simulink model "spe_servomotor_mod"  (R2019a)
settings: Solver=ode23t  StartTime=0.0  StopTime=5  FixedStep=0.001  RelTol=1e-4  EnableMultiTasking=on
model workspace (MAT data in the model file):
  B = 0.000415543589544
  J = 9.65688521823e-08
  Jd = 0.000158042874485
  Km = 0.0648451554932
  La = 0.00823160993738
  Ra = 0.292898808666
  spe_servomotor_mod_spesession : sldodialogs.data.SessionData (value not decoded)
  spe_servomotor_sdosession = sldodialogs.data.SessionData
  spe_servomotor_sdosession.Version = '3.0'
  spe_servomotor_sdosession.Data.ModelName = 'spe_servomotor'
  spe_servomotor_sdosession.Data.ToolType = 'ParameterEstimation'
  spe_servomotor_sdosession.Data.GUIOptions.NoPromptClose = 0
  spe_servomotor_sdosession.Data.Workspace.LocalWorkspace.EstimationData = sdo.Experiment
  spe_servomotor_sdosession.Data.Workspace.LocalWorkspace.EstimationData.ModelName = 'spe_servomotor'
  spe_servomotor_sdosession.Data.Workspace.LocalWorkspace.EstimationData.InputData = Simulink.SimulationData.Signal
  spe_servomotor_sdosession.Data.Workspace.LocalWorkspace.EstimationData.InputData.BlockPath = Simulink.SimulationData.BlockPath
  spe_servomotor_sdosession.Data.Workspace.LocalWorkspace.EstimationData.InputData.BlockPath.path = {'spe_servomotor/Input Signal (V)'}
  spe_servomotor_sdosession.Data.Workspace.LocalWorkspace.EstimationData.InputData.Values = timeseries
  spe_servomotor_sdosession.Data.Workspace.LocalWorkspace.EstimationData.InputData.Values.Name = 'spe_servomotor/Input Signal (V):1'
  spe_servomotor_sdosession.Data.Workspace.LocalWorkspace.EstimationData.InputData.Values.DataInfo = tsdata.datametadata
  spe_servomotor_sdosession.Data.Workspace.LocalWorkspace.EstimationData.InputData.Values.DataInfo.Interpolation = tsdata.interpolation
  spe_servomotor_sdosession.Data.Workspace.LocalWorkspace.EstimationData.InputData.Values.DataInfo.Interpolation.Fhandle : function handle (value not decoded)
  spe_servomotor_sdosession.Data.Workspace.LocalWorkspace.EstimationData.InputData.Values.DataInfo.Interpolation.Name = 'linear'
  spe_servomotor_sdosession.Data.Workspace.LocalWorkspace.EstimationData.InputData.Values.TimeInfo = tsdata.timemetadata
  spe_servomotor_sdosession.Data.Workspace.LocalWorkspace.EstimationData.InputData.Values.TimeInfo.Length = 1001
  spe_servomotor_sdosession.Data.Workspace.LocalWorkspace.EstimationData.InputData.Values.TimeInfo.DuplicateTimes = 0
  spe_servomotor_sdosession.Data.Workspace.LocalWorkspace.EstimationData.InputData.Values.TimeInfo.Time_ = [0 0.005 0.01 0.015 0.02 0.025 0.03 0.035 0.04 0.045 0.05 0.055 ... (1001 elements, 1001x1)]
  spe_servomotor_sdosession.Data.Workspace.LocalWorkspace.EstimationData.InputData.Values.TimeInfo.Initialized = 1
  spe_servomotor_sdosession.Data.Workspace.LocalWorkspace.EstimationData.InputData.Values.QualityInfo = tsdata.qualmetadata
  spe_servomotor_sdosession.Data.Workspace.LocalWorkspace.EstimationData.InputData.Values.Data_ = [1 1 1 1 1 1 1 1 1 1 1 1 ... (1001 elements, 1001x1)]
  spe_servomotor_sdosession.Data.Workspace.LocalWorkspace.EstimationData.InputData.Name = 'spe_servomotor/Input Signal (V):1'
  spe_servomotor_sdosession.Data.Workspace.LocalWorkspace.EstimationData.OutputData = Simulink.SimulationData.Signal
  spe_servomotor_sdosession.Data.Workspace.LocalWorkspace.EstimationData.OutputData.PortType = 'outport'
  spe_servomotor_sdosession.Data.Workspace.LocalWorkspace.EstimationData.OutputData.BlockPath = Simulink.SimulationData.BlockPath
  spe_servomotor_sdosession.Data.Workspace.LocalWorkspace.EstimationData.OutputData.BlockPath.path = {'spe_servomotor/rad to deg'}
  spe_servomotor_sdosession.Data.Workspace.LocalWorkspace.EstimationData.OutputData.Values = timeseries
  spe_servomotor_sdosession.Data.Workspace.LocalWorkspace.EstimationData.OutputData.Values.Name = 'spe_servomotor/rad to deg:1'
  spe_servomotor_sdosession.Data.Workspace.LocalWorkspace.EstimationData.OutputData.Values.DataInfo = tsdata.datametadata
  spe_servomotor_sdosession.Data.Workspace.LocalWorkspace.EstimationData.OutputData.Values.DataInfo.Interpolation = tsdata.interpolation
  spe_servomotor_sdosession.Data.Workspace.LocalWorkspace.EstimationData.OutputData.Values.DataInfo.Interpolation.Fhandle : function handle (value not decoded)
  spe_servomotor_sdosession.Data.Workspace.LocalWorkspace.EstimationData.OutputData.Values.DataInfo.Interpolation.Name = 'linear'
  spe_servomotor_sdosession.Data.Workspace.LocalWorkspace.EstimationData.OutputData.Values.TimeInfo = tsdata.timemetadata
  spe_servomotor_sdosession.Data.Workspace.LocalWorkspace.EstimationData.OutputData.Values.TimeInfo.Length = 1001
  spe_servomotor_sdosession.Data.Workspace.LocalWorkspace.EstimationData.OutputData.Values.TimeInfo.DuplicateTimes = 0
  spe_servomotor_sdosession.Data.Workspace.LocalWorkspace.EstimationData.OutputData.Values.TimeInfo.Time_ = [0 0.005 0.01 0.015 0.02 0.025 0.03 0.035 0.04 0.045 0.05 0.055 ... (1001 elements, 1001x1)]
  spe_servomotor_sdosession.Data.Workspace.LocalWorkspace.EstimationData.OutputData.Values.TimeInfo.Initialized = 1
  spe_servomotor_sdosession.Data.Workspace.LocalWorkspace.EstimationData.OutputData.Values.QualityInfo = tsdata.qualmetadata
  spe_servomotor_sdosession.Data.Workspace.LocalWorkspace.EstimationData.OutputData.Values.Data_ = [2.64853348517 2.69948102795 2.8809816491 3.35224641981 3.98272226171 4.71827741059 5.33283214537 6.22441414402 7.17012790686 7.9534463771 8.97239723269 9.90855833127 ... (1001 elements, 1001x1)]
  spe_servomotor_sdosession.Data.Workspace.LocalWorkspace.EstimationData.OutputData.Name = 'spe_servomotor/rad to deg:1'
  spe_servomotor_sdosession.Data.Workspace.LocalWorkspace.EstimationData.Name = 'EstimationData'
  spe_servomotor_sdosession.Data.Workspace.LocalWorkspace.ValidationData = sdo.Experiment
  spe_servomotor_sdosession.Data.Workspace.LocalWorkspace.ValidationData.ModelName = 'spe_servomotor'
  spe_servomotor_sdosession.Data.Workspace.LocalWorkspace.ValidationData.InputData = Simulink.SimulationData.Signal
  spe_servomotor_sdosession.Data.Workspace.LocalWorkspace.ValidationData.InputData.BlockPath = Simulink.SimulationData.BlockPath
  spe_servomotor_sdosession.Data.Workspace.LocalWorkspace.ValidationData.InputData.BlockPath.path = {'spe_servomotor/Input Signal (V)'}
  spe_servomotor_sdosession.Data.Workspace.LocalWorkspace.ValidationData.InputData.Values = timeseries
  spe_servomotor_sdosession.Data.Workspace.LocalWorkspace.ValidationData.InputData.Values.Name = 'unnamed'
  spe_servomotor_sdosession.Data.Workspace.LocalWorkspace.ValidationData.InputData.Values.DataInfo = tsdata.datametadata
  spe_servomotor_sdosession.Data.Workspace.LocalWorkspace.ValidationData.InputData.Values.DataInfo.Interpolation = tsdata.interpolation
  spe_servomotor_sdosession.Data.Workspace.LocalWorkspace.ValidationData.InputData.Values.DataInfo.Interpolation.Fhandle : function handle (value not decoded)
  spe_servomotor_sdosession.Data.Workspace.LocalWorkspace.ValidationData.InputData.Values.DataInfo.Interpolation.Name = 'linear'
  spe_servomotor_sdosession.Data.Workspace.LocalWorkspace.ValidationData.InputData.Values.TimeInfo = tsdata.timemetadata
  spe_servomotor_sdosession.Data.Workspace.LocalWorkspace.ValidationData.InputData.Values.TimeInfo.Length = 1001
  spe_servomotor_sdosession.Data.Workspace.LocalWorkspace.ValidationData.InputData.Values.TimeInfo.DuplicateTimes = 0
  spe_servomotor_sdosession.Data.Workspace.LocalWorkspace.ValidationData.InputData.Values.TimeInfo.Time_ = [0 0.005 0.01 0.015 0.02 0.025 0.03 0.035 0.04 0.045 0.05 0.055 ... (1001 elements, 1001x1)]
  spe_servomotor_sdosession.Data.Workspace.LocalWorkspace.ValidationData.InputData.Values.TimeInfo.Initialized = 1
  spe_servomotor_sdosession.Data.Workspace.LocalWorkspace.ValidationData.InputData.Values.QualityInfo = tsdata.qualmetadata
  spe_servomotor_sdosession.Data.Workspace.LocalWorkspace.ValidationData.InputData.Values.Data_ = [0 0 0 0 0 0 0 0 0 0 0 0 ... (1001 elements, 1001x1)]
  spe_servomotor_sdosession.Data.Workspace.LocalWorkspace.ValidationData.OutputData = Simulink.SimulationData.Signal
  spe_servomotor_sdosession.Data.Workspace.LocalWorkspace.ValidationData.OutputData.PortType = 'outport'
  spe_servomotor_sdosession.Data.Workspace.LocalWorkspace.ValidationData.OutputData.BlockPath = Simulink.SimulationData.BlockPath
  spe_servomotor_sdosession.Data.Workspace.LocalWorkspace.ValidationData.OutputData.BlockPath.path = {'spe_servomotor/rad to deg'}
  spe_servomotor_sdosession.Data.Workspace.LocalWorkspace.ValidationData.OutputData.Values = timeseries
  spe_servomotor_sdosession.Data.Workspace.LocalWorkspace.ValidationData.OutputData.Values.Name = 'unnamed'
  spe_servomotor_sdosession.Data.Workspace.LocalWorkspace.ValidationData.OutputData.Values.DataInfo = tsdata.datametadata
  spe_servomotor_sdosession.Data.Workspace.LocalWorkspace.ValidationData.OutputData.Values.DataInfo.Interpolation = tsdata.interpolation
  spe_servomotor_sdosession.Data.Workspace.LocalWorkspace.ValidationData.OutputData.Values.DataInfo.Interpolation.Fhandle : function handle (value not decoded)
  spe_servomotor_sdosession.Data.Workspace.LocalWorkspace.ValidationData.OutputData.Values.DataInfo.Interpolation.Name = 'linear'
  spe_servomotor_sdosession.Data.Workspace.LocalWorkspace.ValidationData.OutputData.Values.TimeInfo = tsdata.timemetadata
  spe_servomotor_sdosession.Data.Workspace.LocalWorkspace.ValidationData.OutputData.Values.TimeInfo.Length = 1001
  spe_servomotor_sdosession.Data.Workspace.LocalWorkspace.ValidationData.OutputData.Values.TimeInfo.DuplicateTimes = 0
  spe_servomotor_sdosession.Data.Workspace.LocalWorkspace.ValidationData.OutputData.Values.TimeInfo.Time_ = [0 0.005 0.01 0.015 0.02 0.025 0.03 0.035 0.04 0.045 0.05 0.055 ... (1001 elements, 1001x1)]
  spe_servomotor_sdosession.Data.Workspace.LocalWorkspace.ValidationData.OutputData.Values.TimeInfo.Initialized = 1
  spe_servomotor_sdosession.Data.Workspace.LocalWorkspace.ValidationData.OutputData.Values.QualityInfo = tsdata.qualmetadata
  spe_servomotor_sdosession.Data.Workspace.LocalWorkspace.ValidationData.OutputData.Values.Data_ = [2.6485 2.6485 2.64849999999 2.64849999999 2.64849999999 2.64849999999 2.64849999999 2.64849999999 2.64849999999 2.64849999999 2.64849999999 2.64849999999 ... (1001 elements, 1001x1)]
  spe_servomotor_sdosession.Data.Workspace.LocalWorkspace.ValidationData.Name = 'ValidationData'
  spe_servomotor_sdosession.Data.Workspace.HiddenWorkspace.EstimatedParams(1) = param.Continuous
  spe_servomotor_sdosession.Data.Workspace.HiddenWorkspace.EstimatedParams(1).Minimum_ = 0
  spe_servomotor_sdosession.Data.Workspace.HiddenWorkspace.EstimatedParams(1).Scale_ = 0.008
  spe_servomotor_sdosession.Data.Workspace.HiddenWorkspace.EstimatedParams(1).Size_ = [1 1]
  spe_servomotor_sdosession.Data.Workspace.HiddenWorkspace.EstimatedParams(1).Value_ = 0.008
  spe_servomotor_sdosession.Data.Workspace.HiddenWorkspace.EstimatedParams(1).pID = paramid.Variable
  spe_servomotor_sdosession.Data.Workspace.HiddenWorkspace.EstimatedParams(1).pID.Name = 'B'
  spe_servomotor_sdosession.Data.Workspace.HiddenWorkspace.EstimatedParams(2) = param.Continuous
  spe_servomotor_sdosession.Data.Workspace.HiddenWorkspace.EstimatedParams(2).Minimum_ = 0
  spe_servomotor_sdosession.Data.Workspace.HiddenWorkspace.EstimatedParams(2).Scale_ = 5.7e-07
  spe_servomotor_sdosession.Data.Workspace.HiddenWorkspace.EstimatedParams(2).Size_ = [1 1]
  spe_servomotor_sdosession.Data.Workspace.HiddenWorkspace.EstimatedParams(2).Value_ = 5.7e-07
  spe_servomotor_sdosession.Data.Workspace.HiddenWorkspace.EstimatedParams(2).pID = paramid.Variable
  spe_servomotor_sdosession.Data.Workspace.HiddenWorkspace.EstimatedParams(2).pID.Name = 'J'
  spe_servomotor_sdosession.Data.Workspace.HiddenWorkspace.EstimatedParams(3) = param.Continuous
  spe_servomotor_sdosession.Data.Workspace.HiddenWorkspace.EstimatedParams(3).Minimum_ = 0
  spe_servomotor_sdosession.Data.Workspace.HiddenWorkspace.EstimatedParams(3).Scale_ = 0.0134
  spe_servomotor_sdosession.Data.Workspace.HiddenWorkspace.EstimatedParams(3).Size_ = [1 1]
  spe_servomotor_sdosession.Data.Workspace.HiddenWorkspace.EstimatedParams(3).Value_ = 0.0134
  spe_servomotor_sdosession.Data.Workspace.HiddenWorkspace.EstimatedParams(3).pID = paramid.Variable
  spe_servomotor_sdosession.Data.Workspace.HiddenWorkspace.EstimatedParams(3).pID.Name = 'Km'
  spe_servomotor_sdosession.Data.Workspace.HiddenWorkspace.EstimatedParams(4) = param.Continuous
  spe_servomotor_sdosession.Data.Workspace.HiddenWorkspace.EstimatedParams(4).Minimum_ = 0
  spe_servomotor_sdosession.Data.Workspace.HiddenWorkspace.EstimatedParams(4).Scale_ = 6.5e-05
  spe_servomotor_sdosession.Data.Workspace.HiddenWorkspace.EstimatedParams(4).Size_ = [1 1]
  spe_servomotor_sdosession.Data.Workspace.HiddenWorkspace.EstimatedParams(4).Value_ = 6.5e-05
  spe_servomotor_sdosession.Data.Workspace.HiddenWorkspace.EstimatedParams(4).pID = paramid.Variable
  spe_servomotor_sdosession.Data.Workspace.HiddenWorkspace.EstimatedParams(4).pID.Name = 'La'
  spe_servomotor_sdosession.Data.Workspace.HiddenWorkspace.EstimatedParams(5) = param.Continuous
  spe_servomotor_sdosession.Data.Workspace.HiddenWorkspace.EstimatedParams(5).Minimum_ = 0
  spe_servomotor_sdosession.Data.Workspace.HiddenWorkspace.EstimatedParams(5).Scale_ = 1.9
  spe_servomotor_sdosession.Data.Workspace.HiddenWorkspace.EstimatedParams(5).Size_ = [1 1]
  spe_servomotor_sdosession.Data.Workspace.HiddenWorkspace.EstimatedParams(5).Value_ = 1.9
  spe_servomotor_sdosession.Data.Workspace.HiddenWorkspace.EstimatedParams(5).pID = paramid.Variable
  spe_servomotor_sdosession.Data.Workspace.HiddenWorkspace.EstimatedParams(5).pID.Name = 'Ra'
  spe_servomotor_sdosession.Data.Workspace.HiddenWorkspace.UVars = []
  spe_servomotor_sdosession.Data.ToolData.PlotManager.Plots.Class = 'sldoplots.ExperimentPlot'
  spe_servomotor_sdosession.Data.ToolData.PlotManager.Plots.Sources = {'EstimationData'}
  spe_servomotor_sdosession.Data.ToolData.DialogManager = []
  spe_servomotor_sdosession.Data.ToolData.ParameterEstimation.DesignVariables = 'EstimatedParams'
  spe_servomotor_sdosession.Data.ToolData.ParameterEstimation.UncertainVariables = 'UVars'
  spe_servomotor_sdosession.Data.ToolData.ParameterEstimation.Options = sdo.OptimizeOptions
  spe_servomotor_sdosession.Data.ToolData.ParameterEstimation.Options.Method = 'lsqnonlin'
  spe_servomotor_sdosession.Data.ToolData.ParameterEstimation.Options.MethodOptions.Display = 'iter'
  spe_servomotor_sdosession.Data.ToolData.ParameterEstimation.Options.MethodOptions.MaxFunEvals = 400
  spe_servomotor_sdosession.Data.ToolData.ParameterEstimation.Options.MethodOptions.MaxIter = 100
  spe_servomotor_sdosession.Data.ToolData.ParameterEstimation.Options.MethodOptions.TolFun = 0.2
  spe_servomotor_sdosession.Data.ToolData.ParameterEstimation.Options.MethodOptions.TolX = 1e-06
  spe_servomotor_sdosession.Data.ToolData.ParameterEstimation.Options.MethodOptions.FunValCheck = 'off'
  spe_servomotor_sdosession.Data.ToolData.ParameterEstimation.Options.MethodOptions.OutputFcn = []
  spe_servomotor_sdosession.Data.ToolData.ParameterEstimation.Options.MethodOptions.PlotFcns = []
  spe_servomotor_sdosession.Data.ToolData.ParameterEstimation.Options.MethodOptions.ActiveConstrTol = []
  spe_servomotor_sdosession.Data.ToolData.ParameterEstimation.Options.MethodOptions.Algorithm = 'trust-region-reflective'
  spe_servomotor_sdosession.Data.ToolData.ParameterEstimation.Options.MethodOptions.AlwaysHonorConstraints = []
  spe_servomotor_sdosession.Data.ToolData.ParameterEstimation.Options.MethodOptions.BranchStrategy = []
  spe_servomotor_sdosession.Data.ToolData.ParameterEstimation.Options.MethodOptions.DerivativeCheck = 'off'
  spe_servomotor_sdosession.Data.ToolData.ParameterEstimation.Options.MethodOptions.Diagnostics = 'off'
  spe_servomotor_sdosession.Data.ToolData.ParameterEstimation.Options.MethodOptions.DiffMaxChange = 0.1
  spe_servomotor_sdosession.Data.ToolData.ParameterEstimation.Options.MethodOptions.DiffMinChange = 1e-08
  spe_servomotor_sdosession.Data.ToolData.ParameterEstimation.Options.MethodOptions.FinDiffRelStep = []
  spe_servomotor_sdosession.Data.ToolData.ParameterEstimation.Options.MethodOptions.FinDiffType = 'forward'
  spe_servomotor_sdosession.Data.ToolData.ParameterEstimation.Options.MethodOptions.GoalsExactAchieve = []
  spe_servomotor_sdosession.Data.ToolData.ParameterEstimation.Options.MethodOptions.GradConstr = []
  spe_servomotor_sdosession.Data.ToolData.ParameterEstimation.Options.MethodOptions.GradObj = []
  spe_servomotor_sdosession.Data.ToolData.ParameterEstimation.Options.MethodOptions.HessFcn = []
  spe_servomotor_sdosession.Data.ToolData.ParameterEstimation.Options.MethodOptions.Hessian = []
  spe_servomotor_sdosession.Data.ToolData.ParameterEstimation.Options.MethodOptions.HessMult = []
  spe_servomotor_sdosession.Data.ToolData.ParameterEstimation.Options.MethodOptions.HessPattern = []
  spe_servomotor_sdosession.Data.ToolData.ParameterEstimation.Options.MethodOptions.HessUpdate = []
  spe_servomotor_sdosession.Data.ToolData.ParameterEstimation.Options.MethodOptions.InitialHessType = []
  spe_servomotor_sdosession.Data.ToolData.ParameterEstimation.Options.MethodOptions.InitialHessMatrix = []
  spe_servomotor_sdosession.Data.ToolData.ParameterEstimation.Options.MethodOptions.InitBarrierParam = []
  spe_servomotor_sdosession.Data.ToolData.ParameterEstimation.Options.MethodOptions.InitTrustRegionRadius = []
  spe_servomotor_sdosession.Data.ToolData.ParameterEstimation.Options.MethodOptions.Jacobian = 'on'
  spe_servomotor_sdosession.Data.ToolData.ParameterEstimation.Options.MethodOptions.JacobMult = []
  spe_servomotor_sdosession.Data.ToolData.ParameterEstimation.Options.MethodOptions.JacobPattern = 'sparse(ones(jrows,jcols))'
  spe_servomotor_sdosession.Data.ToolData.ParameterEstimation.Options.MethodOptions.LargeScale = []
  spe_servomotor_sdosession.Data.ToolData.ParameterEstimation.Options.MethodOptions.MaxNodes = []
  spe_servomotor_sdosession.Data.ToolData.ParameterEstimation.Options.MethodOptions.MaxPCGIter = 'max(1,floor(numberofvariables/2))'
  spe_servomotor_sdosession.Data.ToolData.ParameterEstimation.Options.MethodOptions.MaxProjCGIter = []
  spe_servomotor_sdosession.Data.ToolData.ParameterEstimation.Options.MethodOptions.MaxRLPIter = []
  spe_servomotor_sdosession.Data.ToolData.ParameterEstimation.Options.MethodOptions.MaxSQPIter = []
  spe_servomotor_sdosession.Data.ToolData.ParameterEstimation.Options.MethodOptions.MaxTime = []
  spe_servomotor_sdosession.Data.ToolData.ParameterEstimation.Options.MethodOptions.MeritFunction = []
  spe_servomotor_sdosession.Data.ToolData.ParameterEstimation.Options.MethodOptions.MinAbsMax = []
  spe_servomotor_sdosession.Data.ToolData.ParameterEstimation.Options.MethodOptions.NodeDisplayInterval = []
  spe_servomotor_sdosession.Data.ToolData.ParameterEstimation.Options.MethodOptions.NodeSearchStrategy = []
  spe_servomotor_sdosession.Data.ToolData.ParameterEstimation.Options.MethodOptions.NoStopIfFlatInfeas = []
  spe_servomotor_sdosession.Data.ToolData.ParameterEstimation.Options.MethodOptions.ObjectiveLimit = []
  spe_servomotor_sdosession.Data.ToolData.ParameterEstimation.Options.MethodOptions.PhaseOneTotalScaling = []
  spe_servomotor_sdosession.Data.ToolData.ParameterEstimation.Options.MethodOptions.Preconditioner = []
  spe_servomotor_sdosession.Data.ToolData.ParameterEstimation.Options.MethodOptions.PrecondBandWidth = Inf
  spe_servomotor_sdosession.Data.ToolData.ParameterEstimation.Options.MethodOptions.RelLineSrchBnd = []
  spe_servomotor_sdosession.Data.ToolData.ParameterEstimation.Options.MethodOptions.RelLineSrchBndDuration = []
  spe_servomotor_sdosession.Data.ToolData.ParameterEstimation.Options.MethodOptions.ScaleProblem = 'none'
  spe_servomotor_sdosession.Data.ToolData.ParameterEstimation.Options.MethodOptions.Simplex = []
  spe_servomotor_sdosession.Data.ToolData.ParameterEstimation.Options.MethodOptions.SubproblemAlgorithm = []
  spe_servomotor_sdosession.Data.ToolData.ParameterEstimation.Options.MethodOptions.TolCon = 0.001
  spe_servomotor_sdosession.Data.ToolData.ParameterEstimation.Options.MethodOptions.TolConSQP = []
  spe_servomotor_sdosession.Data.ToolData.ParameterEstimation.Options.MethodOptions.TolGradCon = []
  spe_servomotor_sdosession.Data.ToolData.ParameterEstimation.Options.MethodOptions.TolPCG = 0.1
  spe_servomotor_sdosession.Data.ToolData.ParameterEstimation.Options.MethodOptions.TolProjCG = []
  spe_servomotor_sdosession.Data.ToolData.ParameterEstimation.Options.MethodOptions.TolProjCGAbs = []
  spe_servomotor_sdosession.Data.ToolData.ParameterEstimation.Options.MethodOptions.TolRLPFun = []
  spe_servomotor_sdosession.Data.ToolData.ParameterEstimation.Options.MethodOptions.TolXInteger = []
  spe_servomotor_sdosession.Data.ToolData.ParameterEstimation.Options.MethodOptions.TypicalX = 'ones(numberofvariables,1)'
  spe_servomotor_sdosession.Data.ToolData.ParameterEstimation.Options.MethodOptions.UseParallel = 'never'
  spe_servomotor_sdosession.Data.ToolData.ParameterEstimation.Options.OptimizedModel = 'spe_servomotor'
  spe_servomotor_sdosession.Data.ToolData.ParameterEstimation.GUIOptions.ShowProgress = 1
  spe_servomotor_sdosession.Data.ToolData.ParameterEstimation.GUIOptions.UpdatePlots = 1
  spe_servomotor_sdosession.Data.ToolData.ParameterEstimation.GUIOptions.UpdateModel = 1
  spe_servomotor_sdosession.Data.ToolData.ParameterEstimation.GUIOptions.UpdateDesign = 'overwrite'
  spe_servomotor_sdosession.Data.ToolData.ParameterEstimation.GUIOptions.SaveReport = 0
  spe_servomotor_sdosession.Data.ToolData.ParameterEstimation.GUIOptions.SaveRequirementValue = 1
  spe_servomotor_sdosession.Data.ToolData.ParameterEstimation.DataToPlot = ''
  spe_servomotor_sdosession.Data.ToolData.ParameterEstimation.LocalRequirements = struct([])
  spe_servomotor_sdosession.Data.ToolData.ParameterEstimation.BlockRequirements = struct([])
  spe_servomotor_sdosession.Data.ToolData.ParameterEstimation.LocalExperiments(1).SelectedForEstimation = 1
  spe_servomotor_sdosession.Data.ToolData.ParameterEstimation.LocalExperiments(1).SelectedForValidation = 0
  spe_servomotor_sdosession.Data.ToolData.ParameterEstimation.LocalExperiments(1).Experiment = 'EstimationData'
  spe_servomotor_sdosession.Data.ToolData.ParameterEstimation.LocalExperiments(2).SelectedForEstimation = 0
  spe_servomotor_sdosession.Data.ToolData.ParameterEstimation.LocalExperiments(2).SelectedForValidation = 0
  spe_servomotor_sdosession.Data.ToolData.ParameterEstimation.LocalExperiments(2).Experiment = 'ValidationData'
  spe_servomotor_sdosession.Data.ToolData.ParameterEstimation.LocalResults.SelectedForValidation = 1
  spe_servomotor_sdosession.Data.ToolData.ParameterEstimation.LocalResults.Result = 'Use current parameter values'
  spe_servomotor_sdosession.Data.ToolData.ParameterEstimation.Cost.Type = 'SSE'
  spe_servomotor_sdosession.Data.ToolData.ParameterEstimation.Cost.Robust = 'off'
  x0 = 2.6485
undefined symbols (not defined in the file or in its folder): sigbuilder_block
libraries: fl_lib x16, nesl_utility x7, ee_lib x4, fl_ps_legacy_lib x2, simulink x2
settings Model: OrderedModelArguments=off  Creator=The MathWorks, Inc.  LastModifiedBy=kalyan
settings SolverCC: SolverResetMethod=Robust
settings DataIOCC: SaveFormat=Array  SaveOutput=off  SignalLogging=off  SaveTime=off  ReturnWorkspaceOutputs=off
settings OptimizationCC: ExpressionDepthLimit=2147483647  InitFltsAndDblsToZero=on  LifeSpan=1
settings DebuggingCC: AlgebraicLoopMsg=none  ArtificialAlgebraicLoopMsg=none  SaveWithParameterizedLinksMsg=none  UnderspecifiedInitializationDetection=Classic  MergeDetectMultiDrivingBlocksExec=none  SignalResolutionControl=TryResolveAllWithWarning  MultiTaskDSMMsg=warning  MultiTaskCondExecSysMsg=none  FcnCallInpInsideContextMsg=warning  AllowSymbolicDim=off  StateNameClashWarn=warning  SFUnexpectedBacktrackingDiag=warning  SFNoUnconditionalDefaultTransitionDiag=warning  SFExecutionAtInitializationDiag=none  ArithmeticOperatorsInVariantConditions=warning
settings HardwareCC: ProdBitPerPointer=32  ProdBitPerSizeT=32  ProdBitPerPtrDiffT=32  ProdLargestAtomicFloat=None  ProdIntDivRoundTo=Undefined  ProdEndianess=Unspecified  ProdWordSize=32  ProdHWDeviceType=32-bit Generic
settings ModelReferenceCC: PropagateSignalLabelsOutOfModel=off
settings SFSimCC: SimUseLocalCustomCode=off  SimParseCustomCode=off  MATLABDynamicMemAlloc=off
settings RTWCC: SystemTargetFile=ert.tlc  GenCodeOnly=on  TemplateMakefile=ert_default_tmf  Description=RTW Embedded Coder (no auto configuration)  RTWUseLocalCustomCode=off
settings CodeAppCC: IgnoreCustomStorageClasses=off  CustomSymbolStrType=$N$R$M  StateflowObjectComments=on  InternalIdentifier=Classic
settings ERTTargetCC: TargetFcnLib=ansi_tfl_tmw.mat  MultiwordLength=2048  GenerateSampleERTMain=on  SupportContinuousTime=on  SupportNonInlinedSFcns=on  ERTCustomFileTemplate=example_file_process.tlc  ConvertIfToSwitch=off  SuppressUnreachableDefaultCases=off
settings ConfigComp: CovMetricSettings=dw  CovHtmlReporting=on  CovSaveCumulativeToWorkspaceVar=on  CovSaveSingleToWorkspaceVar=on  CovExternalEMLEnable=off  CovSFcnEnable=off
settings SimscapeCC: SimscapeNormalizeSystem=off

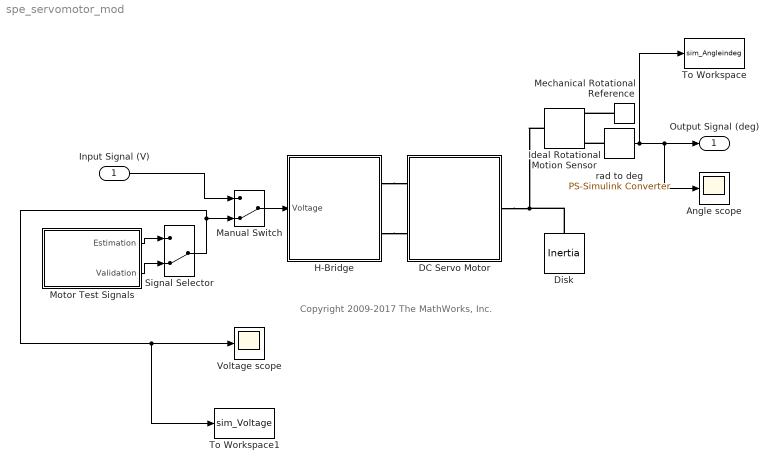
== system spe_servomotor_mod ==
  note: Copyright 2009-2017 The MathWorks, Inc.
  Input Signal (V) : Inport
  Angle scope : Scope
  DC Servo Motor : Subsystem
      mask Display: image('spe_servomotor_motor.jpg')
  Disk : fl_lib/Mechanical/Rotational Elements/Inertia  inertia=Jd kg*m^2  w_specify=off  w_priority=Low  w=0 rad/s  w_nominal_specify=off  w_nominal_unit=rad/s  w_nominal_value=1  t_specify=off  t_priority=None  t=0 N*m  t_nominal_specify=off  t_nominal_unit=N*m  t_nominal_value=1
  H-Bridge : Subsystem
      mask Display: image('spe_servomotor_hbridge.jpg')
  Ideal Rotational Motion Sensor : fl_lib/Mechanical/Mechanical Sensors/Ideal Rotational Motion Sensor  offset=x0*pi/180 rad
  Manual Switch : ManualSwitch  CurrentSetting=0
  Mechanical Rotational Reference : fl_lib/Mechanical/Rotational Elements/Mechanical Rotational Reference
  Motor Test Signals : Subsystem  Tag=STV Subsys  LoadFcn=sigbuilder_block('load',[211.5 0 813 450.75 ]);  StartFcn=sigbuilder_block('start');  StopFcn=sigbuilder_block('stop');  ClipboardFcn=sigbuilder_block('clipboard');  mask(Sigbuilder block){tuvar=[0:10]}
      mask help: Sigbuilder GUI
      mask init:
      | if ~strcmp(get_param(bdroot(gcbh),'SimulationStatus'),'stopped') tuvar = sigbuilder_block('maskInit'); end
      settings: CopyFcn=sigbuilder_block('copy');  DeleteFcn=sigbuilder_block('delete');  ModelCloseFcn=sigbuilder_block('modelClose');  PreSaveFcn=sigbuilder_block('preSave');  PauseFcn=sigbuilder_block('pause')  ContinueFcn=sigbuilder_block('continue')  NameChangeFcn=sigbuilder_block('namechange');  OpenFcn=sigbuilder_block('open',[1100.25 -38.25 813 492 ]);  CloseFcn=sigbuilder_block('close');
      mask Display: plot(0, 0, 100, 100,[2, 2, 32, 32, 2], [68, 8, 8, 68, 68],[32, 2], [38, 38], [32, 19, 2],[53, 60, 44], [32, 17, 17, 2],[16, 16, 31, 31]);txt = getActiveGroup(gcbh);text(2, 100, txt,'verticalAlignment', 'top');
  Signal Selector : ManualSwitch  CurrentSetting=0
  To Workspace : ToWorkspace  VariableName=sim_Angleindeg  SaveFormat=Timeseries  SampleTime=-1
  To Workspace1 : ToWorkspace  VariableName=sim_Voltage  SaveFormat=Timeseries  SampleTime=-1
  Voltage scope : Scope
  rad to deg : nesl_utility/PS-Simulink Converter  PhysicalDomain=network_engine_domain  SubClassName=ps_output  LeftPortType=input  RightPortType=output  PseudoPeriodic=off  Frequencies=[]  Unit=deg  AffineConversion=off
  Output Signal (deg) : Outport
  wires:
  Input Signal (V)/1 -> Manual Switch/1
  Manual Switch/1 -> H-Bridge/1(Voltage)
  Motor Test Signals/1(Estimation) -> Signal Selector/1
  Motor Test Signals/2(Validation) -> Signal Selector/2
  Signal Selector/1 -> To Workspace1/1, Voltage scope/1, Manual Switch/2
  rad to deg/1 -> To Workspace/1, Output Signal (deg)/1, Angle scope/1
  connections:
  Disk/LConn1 -- DC Servo Motor/RConn1 -- Ideal Rotational Motion Sensor/LConn1
  Mechanical Rotational Reference/LConn1 -- Ideal Rotational Motion Sensor/RConn1
  rad to deg/LConn1 -- Ideal Rotational Motion Sensor/RConn3
  H-Bridge/RConn1 -- DC Servo Motor/LConn1
  H-Bridge/RConn2 -- DC Servo Motor/LConn2

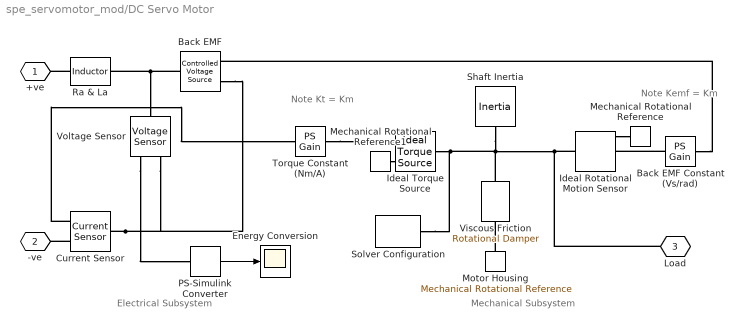
== system spe_servomotor_mod/DC Servo Motor ==
  note: Electrical
      | Subsystem
  note: Mechanical
      | Subsystem
  note: Note
      | Kt = Km
  note: Note
      | Kemf = Km
  Back EMF : fl_lib/Electrical/Electrical Sources/Controlled Voltage Source
  Back EMF Constant (Vs/rad) : fl_ps_legacy_lib/Legacy Physical Signals/Functions/PS Gain  gain=Km
      settings: SourceProductName=Simscape
  Current Sensor : fl_lib/Electrical/Electrical Sensors/Current Sensor
  Energy Conversion : Scope
  Ideal Rotational Motion Sensor : fl_lib/Mechanical/Mechanical Sensors/Ideal Rotational Motion Sensor  offset=x0*pi/180 rad
  Ideal Torque Source : fl_lib/Mechanical/Mechanical Sources/Ideal Torque Source
  Mechanical Rotational Reference : fl_lib/Mechanical/Rotational Elements/Mechanical Rotational Reference
  Mechanical Rotational Reference1 : fl_lib/Mechanical/Rotational Elements/Mechanical Rotational Reference
  Motor Housing : fl_lib/Mechanical/Rotational Elements/Mechanical Rotational Reference
  PS-Simulink Converter : nesl_utility/PS-Simulink Converter  PhysicalDomain=network_engine_domain  SubClassName=ps_output  LeftPortType=input  RightPortType=output  PseudoPeriodic=off  Frequencies=[]  Unit=1  AffineConversion=off
  Ra & La : fl_lib/Electrical/Electrical Elements/Inductor  l=La H  r=Ra Ohm  g=0 1/Ohm  i_specify=off  i_priority=None  i=0 A  i_nominal_specify=off  i_nominal_unit=A  i_nominal_value=1  v_specify=off  v_priority=None  v=0 V  v_nominal_specify=off  v_nominal_unit=V  v_nominal_value=1  i_L_specify=off  i_L_priority=High  i_L=0 A  i_L_nominal_specify=off  i_L_nominal_unit=A  i_L_nominal_value=1
  Shaft Inertia : fl_lib/Mechanical/Rotational Elements/Inertia  inertia=J kg*m^2  w_specify=off  w_priority=High  w=0 rad/s  w_nominal_specify=off  w_nominal_unit=rad/s  w_nominal_value=1  t_specify=off  t_priority=None  t=0 N*m  t_nominal_specify=off  t_nominal_unit=N*m  t_nominal_value=1
  Solver Configuration : nesl_utility/Solver Configuration  PhysicalDomain=network_engine_domain  SubClassName=solver  LeftPortType=input  RightPortType=generic  Tones=[]  Harmonics=[]  SimulateNoise=off  Profile=off  UseLocalSampling=off  EnableSwitchedLinearOptims=on  FrequencyDomain=off  UseCCode=off  RelTol=0.001  AbsTol=1e-06  MinStep=1e-09  ToWorkspace=off  RevertToSquareIcSolve=off  NumHomotopyIterations=100  PhasorMode=off  PhasorModeNumHarmonics=1  DoDC=off  ResidualTolerance=1e-9  UseLocalSolver=off  LocalSolverChoice=NE_BACKWARD_EULER_ADVANCER  LocalSolverSampleTime=.001  DoFixedCost=off  MaxNonlinIter=3  MaxModeIter=2  LinearAlgebra=Sparse  EquationFormulation=NE_TIME_EF  DelaysMemoryBudget=1024  AutomaticFiltering=on  FilteringTimeConstant=0.001  PartitionStorageMethod=AS_NEEDED  PartitionMemoryBudget=1024  PartitionMethod=FAST
  Torque Constant (Nm/A) : fl_ps_legacy_lib/Legacy Physical Signals/Functions/PS Gain  gain=Km
      settings: SourceProductName=Simscape
  Viscous Friction : fl_lib/Mechanical/Rotational Elements/Rotational Damper  D=B N*m/(rad/s)  w_specify=off  w_priority=None  w=0 rad/s  w_nominal_specify=off  w_nominal_unit=rad/s  w_nominal_value=1  t_specify=off  t_priority=None  t=0 N*m  t_nominal_specify=off  t_nominal_unit=N*m  t_nominal_value=1
  Voltage Sensor : fl_lib/Electrical/Electrical Sensors/Voltage Sensor
  +ve : PMIOPort  Tag=PMCPort  Side=Left
  -ve : PMIOPort  Tag=PMCPort  Port=2  Side=Left
  Load : PMIOPort  Port=3  Side=Right
  wires:
  PS-Simulink Converter/1 -> Energy Conversion/1
  connections:
  Ra & La/LConn1 -- +ve/RConn1
  Viscous Friction/RConn1 -- Ideal Rotational Motion Sensor/LConn1 -- Load/RConn1 -- Shaft Inertia/LConn1 -- Ideal Torque Source/LConn1 -- Solver Configuration/RConn1
  Motor Housing/LConn1 -- Viscous Friction/LConn1
  Back EMF Constant (Vs/rad)/LConn1 -- Ideal Rotational Motion Sensor/RConn2
  Ideal Rotational Motion Sensor/RConn1 -- Mechanical Rotational Reference/LConn1
  Mechanical Rotational Reference1/LConn1 -- Ideal Torque Source/RConn2
  Torque Constant (Nm/A)/RConn1 -- Ideal Torque Source/RConn1
  Back EMF/LConn1 -- Voltage Sensor/LConn1 -- Ra & La/RConn1
  Current Sensor/LConn1 -- Back EMF/RConn2 -- Voltage Sensor/RConn2
  Current Sensor/RConn2 -- -ve/RConn1
  Current Sensor/RConn1 -- Torque Constant (Nm/A)/LConn1
  Back EMF Constant (Vs/rad)/RConn1 -- Back EMF/RConn1
  Voltage Sensor/RConn1 -- PS-Simulink Converter/LConn1

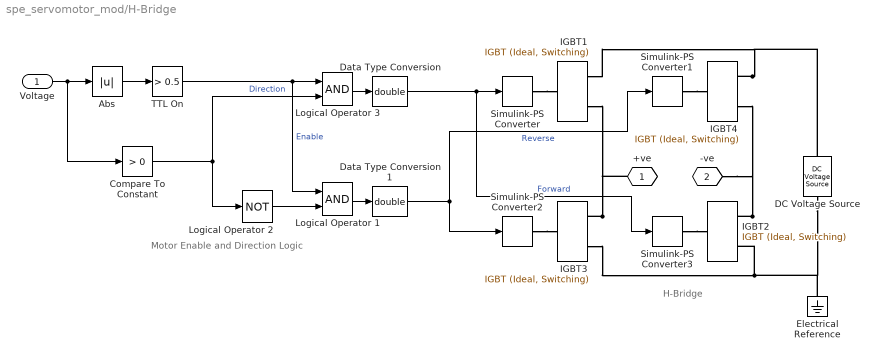
== system spe_servomotor_mod/H-Bridge ==
  note: Motor Enable and Direction Logic
  note: H-Bridge
  Voltage : Inport
  Abs : Abs
  Compare To Constant : simulink/Logic and Bit Operations/Compare To Constant  relop=>  const=0  OutDataTypeStr=boolean  ZeroCross=off
  DC Voltage Source : fl_lib/Electrical/Electrical Sources/DC Voltage Source  v0=6.2 V
  Data Type Conversion : DataTypeConversion  OutDataTypeStr=double
  Data Type Conversion1 : DataTypeConversion  OutDataTypeStr=double
  Electrical Reference : fl_lib/Electrical/Electrical Elements/Electrical Reference
  IGBT{1..4} (4 alike) : ee_lib/Semiconductors & Converters/IGBT (Ideal, Switching)  Vf=1 V  Ron=0.001 Ohm  Goff=1e-5 1/Ohm  Vth=0.5 V  diode_param=1  diode_Vf=0.8 V  diode_Ron=0.001 Ohm  diode_Goff=1e-5 1/Ohm  diode_C=5e-8 F  diode_iRM=-235 A  diode_iF=300 A  diode_idot=-50 A/us  diode_trr_param=1  diode_trr_factor=3  diode_trr=15 us  diode_Qrr=1.5e+3 s*uA  thermal_loss_option=2  Voff=300 V  Tau=1e-4 s  Tj=[298.15, 398.15] K  Iout_scalar=600 A  Eon_scalar=22.86e-3 J  Eoff_scalar=17.14e-3 J  Von_scalar=2.7 V  Iout_data=[0, 10, 50, 100, 200, 400, 600] A  Eon_data=[0, .29, 1.43, 2.86, 5.71, 13.14, 22.86; 0, .57, 2.63, 5.14, 10.29, 20.57, 30.29] * 1e-3 J  Eoff_data=[0, .21, 1.07, 2.14, 4.29, 9.86, 17.14; 0, .43, 1.97, 3.86, 7.71, 15.43, 22.71] * 1e-3 J  Von_data=[0, 1.1, 1.3, 1.45, 1.75, 2.25, 2.7; 0, 1, 1.15, 1.35, 1.7, 2.35, 3] V
      settings: SourceProductName=Simscape Electrical
  Logical Operator 1 : Logic  AllPortsSameDT=off  OutDataTypeStr=boolean
  Logical Operator 2 : Logic  Operator=NOT  AllPortsSameDT=off  OutDataTypeStr=boolean
  Logical Operator 3 : Logic  AllPortsSameDT=off  OutDataTypeStr=boolean
  Simulink-PS Converter{,1..3} (4 alike) : nesl_utility/Simulink-PS Converter  PhysicalDomain=network_engine_domain  SubClassName=ps_input  LeftPortType=input  RightPortType=output  PseudoPeriodic=off  Frequencies=[]  NoiseDistribution=none  NoiseParameters=[]  Unit=1  AffineConversion=off  FilteringAndDerivatives=provide  SimscapeFilterOrder=1  InputFilterTimeConstant=0.001  UdotUserProvided=0
  TTL On : simulink/Logic and Bit Operations/Compare To Constant  relop=>  const=0.5  OutDataTypeStr=boolean  ZeroCross=off
  +ve : PMIOPort  Tag=PMCPort  Side=Right
  -ve : PMIOPort  Tag=PMCPort  Port=2  Side=Right
  wires:
  Data Type Conversion1/1 -> Simulink-PS Converter1/1, Simulink-PS Converter2/1  "Reverse"
  Data Type Conversion/1 -> Simulink-PS Converter3/1, Simulink-PS Converter/1  "Forward"
  Abs/1 -> TTL On/1
  TTL On/1 -> Logical Operator 3/1, Logical Operator 1/1  "Enable"
  Voltage/1 -> Abs/1, Compare To Constant/1
  Compare To Constant/1 -> Logical Operator 3/2, Logical Operator 2/1  "Direction"
  Logical Operator 2/1 -> Logical Operator 1/2
  Logical Operator 3/1 -> Data Type Conversion/1
  Logical Operator 1/1 -> Data Type Conversion1/1
  connections:
  Simulink-PS Converter/RConn1 -- IGBT1/LConn1
  Simulink-PS Converter1/RConn1 -- IGBT4/LConn1
  Simulink-PS Converter2/RConn1 -- IGBT3/LConn1
  Simulink-PS Converter3/RConn1 -- IGBT2/LConn1
  IGBT4/RConn1 -- IGBT1/RConn1 -- DC Voltage Source/LConn1
  IGBT3/RConn1 -- IGBT1/RConn2 -- +ve/RConn1
  IGBT3/RConn2 -- IGBT2/RConn2 -- DC Voltage Source/RConn1 -- Electrical Reference/LConn1
  IGBT2/RConn1 -- IGBT4/RConn2 -- -ve/RConn1

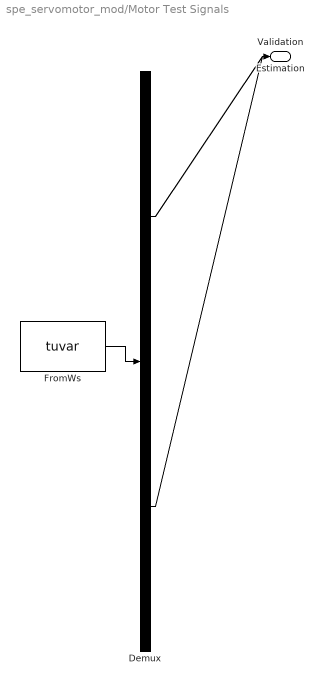
== system spe_servomotor_mod/Motor Test Signals ==
  Demux : Demux  Tag=STV Demux  Outputs=2
  FromWs : FromWorkspace  Tag=STV FromWs  VariableName=tuvar  SampleTime=0
      SigBuilderData=|
      | dataSet.timeRange = [0 5]
      | dataSet.name = 'Test Signals'
      | sbobj.Groups.Name = 'Test Signals'
      | sbobj.Groups.Signals(1).Name = 'Estimation'
      | sbobj.Groups.Signals(1).XData = [0 0.25 0.25 0.5 0.5 0.75 0.75 1 1 1.25 1.25 1.5 1.5 1.75 1.75 2 2 2.25 2.25 2.5 2.5 2.75 2.75 3 3 3.25 3.25 3.5 3.5 3.75 3.75 4 4 4.25 4.25 4.5 4.5 4.75 4.75 5]
      | sbobj.Groups.Signals(1).YData = [3 3 -3 -3 3 3 -3 -3 3 3 -3 -3 3 3 -3 -3 3 3 -3 -3 3 3 -3 -3 3 3 -3 -3 3 3 -3 -3 3 3 -3 -3 3 3 -3 -3]
      | sbobj.Groups.Signals(2).Name = 'Validation'
      | sbobj.Groups.Signals(2).XData = [0 0.75 0.75 1 1 1.5 1.5 1.75 1.75 5]
      | sbobj.Groups.Signals(2).YData = [0 0 3 3 -3 -3 3 3 0 0]
      | sbobj.Groups.TimeRange = [0 5]
  Estimation : Outport  Tag=STV Outport
  Validation : Outport  Tag=STV Outport  Port=2
  wires:
  FromWs/1 -> Demux/1
  Demux/1 -> Estimation/1
  Demux/2 -> Validation/1
